simulink subsystem "PrimitiveBattery_refsub_OLD"  (R2026a)
settings: Solver=VariableStepAuto
undefined symbols (not defined in the file): batteryHV
libraries: fl_lib x9
settings Model: Creator=isaacito  LastModifiedBy=isaacito
settings SimscapeCC: SimscapeNominalValues="[{\"value\":\"1\",\"unit\":\"A\"},{\"value\":\"1\",\"unit\":\"bar\"},{\"value\":\"1\",\"unit\":\"cm^2\"},{\"value\":\"1\",\"unit\":\"cm^3/s\"},{\"value\":\"1\",\"unit\":\"kJ/kg\"},{\"value\":\"1\",\"unit\":\"kW\"},{\"value\":\"1\",\"unit\":\"l\"},{\"value\":\"1\",\"unit\":\"N\"},{\"value\":\"1\",\"unit\":\"N*m\"},{\"value\":\"1\",\"unit\":\"V\"}]"  SimscapeLogType=none  SimscapeLogDataHistory=5000.0

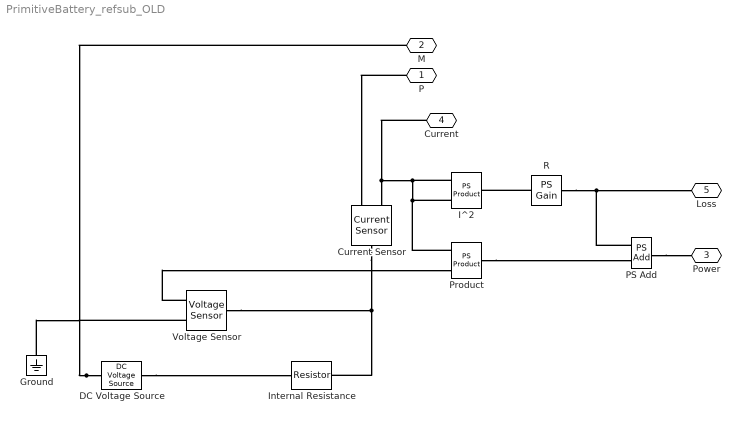
== system PrimitiveBattery_refsub_OLD ==
  Current Sensor : fl_lib/Electrical/Electrical Sensors/Current Sensor
  DC Voltage Source : fl_lib/Electrical/Electrical Sources/DC Voltage Source  v0=batteryHV.nominalVoltage_V V
      settings: AttributesFormatString=%<v0> [%<v0_unit>]
  Ground : fl_lib/Electrical/Electrical Elements/Electrical Reference
  I^2 : fl_lib/Physical Signals/Functions/PS Product
  Internal Resistance : fl_lib/Electrical/Electrical Elements/Resistor  R=batteryHV.internalResistance_Ohm Ohm  i_specify=off  i_priority=High  i=0 A  i_nominal_specify=off  i_nominal_value=1  i_nominal_unit=A  v_specify=off  v_priority=High  v=0 V  v_nominal_specify=off  v_nominal_value=1  v_nominal_unit=V
      settings: AttributesFormatString=%<R> [%<R_unit>]
  PS Add : fl_lib/Physical Signals/Functions/PS Add
  Product : fl_lib/Physical Signals/Functions/PS Product
  R : fl_lib/Physical Signals/Functions/PS Gain  gain=batteryHV.internalResistance_Ohm Ohm
      settings: AttributesFormatString=%<gain> [%<gain_unit>]
  Voltage Sensor : fl_lib/Electrical/Electrical Sensors/Voltage Sensor
  P : PMIOPort  Side=Right
  M : PMIOPort  Port=2  Side=Right
  Power : PMIOPort  Port=3  Side=Right
  Current : PMIOPort  Port=4  Side=Right
  Loss : PMIOPort  Port=5  Side=Right
  connections:
  DC Voltage Source/RConn1 -- Ground/LConn1 -- M/RConn1 -- Voltage Sensor/RConn2
  P/RConn1 -- Current Sensor/RConn2
  Current Sensor/LConn1 -- Voltage Sensor/LConn1 -- Internal Resistance/RConn1
  DC Voltage Source/LConn1 -- Internal Resistance/LConn1
  Voltage Sensor/RConn1 -- Product/LConn1
  Current/RConn1 -- Current Sensor/RConn1 -- I^2/LConn2 -- I^2/LConn1 -- Product/LConn2
  PS Add/LConn1 -- Loss/RConn1 -- R/RConn1
  Product/RConn1 -- PS Add/LConn2
  PS Add/RConn1 -- Power/RConn1
  R/LConn1 -- I^2/RConn1
